simulink model "rendezvous_optimization_ALO"  (R2023a)
settings: Solver=VariableStepAuto  StartTime=0.0  StopTime=600  RelTol=1e-3
undefined symbols (not defined in the file): Ax, Ax_i, Ay, Ay_i, Az, Bx, Bx_i, By, By_i, Bz, Cx, Cx_i, Cy, Cy_i, Cz, IC_x_init, IC_y_init, juliandate, m0, mDot, OC_x_init, OC_y_init, OC_z_init, omega_T, Ve
(part 1 of 2)
settings Model: Creator=shubi  LastModifiedBy=shubi
settings SolverCC: ZeroCrossAlgorithm=Adaptive
settings DebuggingCC: AlgebraicLoopMsg=none  IgnoredZcDiagnostic=none

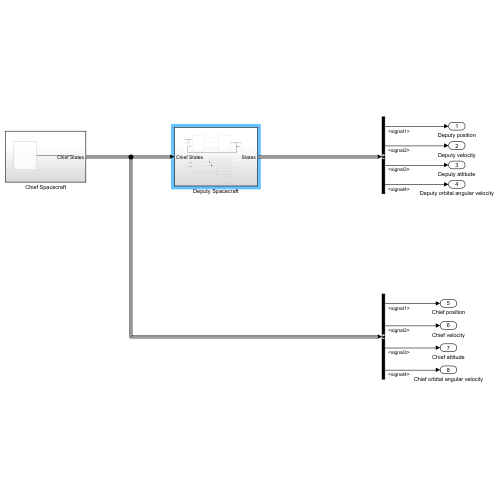
[thumbnail: Simulink's stored preview of the top-level diagram]
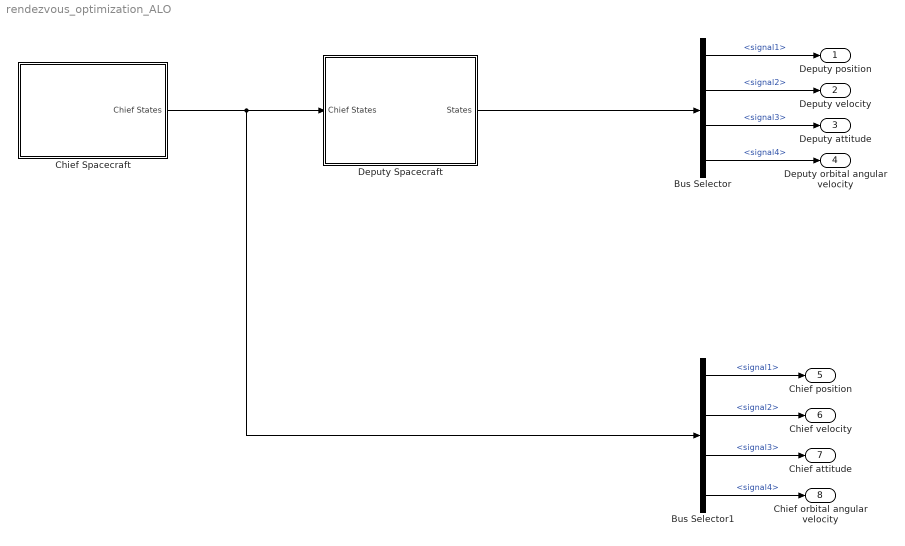
== system rendezvous_optimization_ALO ==
  Bus Selector : BusSelector  OutputSignals=signal1,signal2,signal3,signal4
  Bus Selector1 : BusSelector  OutputSignals=signal1,signal2,signal3,signal4
  Chief Spacecraft : Subsystem
  Deputy Spacecraft : Subsystem
  Deputy position : Outport
  Deputy velocity : Outport  Port=2
  Deputy attitude : Outport  Port=3
  Deputy orbital angular velocity : Outport  Port=4
  Chief position : Outport  Port=5
  Chief velocity : Outport  Port=6
  Chief attitude : Outport  Port=7
  Chief orbital angular velocity : Outport  Port=8
  wires:
  Bus Selector/4 -> Deputy orbital angular velocity/1  "<signal4>"
  Bus Selector1/4 -> Chief orbital angular velocity/1  "<signal4>"
  Bus Selector1/3 -> Chief attitude/1  "<signal3>"
  Bus Selector/2 -> Deputy velocity/1  "<signal2>"
  Bus Selector1/2 -> Chief velocity/1  "<signal2>"
  Bus Selector1/1 -> Chief position/1  "<signal1>"
  Chief Spacecraft/1(Chief States) -> Bus Selector1/1, Deputy Spacecraft/1(Chief States)
  Bus Selector/3 -> Deputy attitude/1  "<signal3>"
  Deputy Spacecraft/1(States) -> Bus Selector/1
  Bus Selector/1 -> Deputy position/1  "<signal1>"

== system rendezvous_optimization_ALO/Chief Spacecraft ==
  Spacecraft : Subsystem
  Chief States : Outport
  wires:
  Spacecraft/1(States) -> Chief States/1

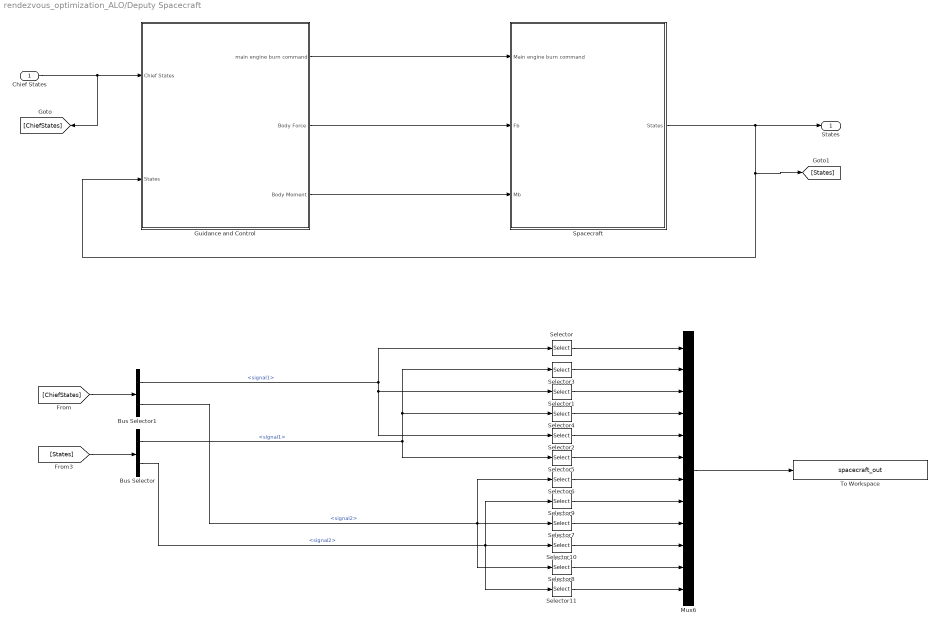
== system rendezvous_optimization_ALO/Deputy Spacecraft ==
  Chief States : Inport
  Bus Selector : BusSelector  OutputSignals=signal1,signal2
  Bus Selector1 : BusSelector  OutputSignals=signal1,signal2
  Guidance and Control : Subsystem
  Mux6 : Mux  Inputs=12
  Selector{,3,6,9} (4 alike) : Selector  InputPortWidth=3  IndexOptions=Index vector (dialog)  Indices=[1]  OutputSizes=1
  Selector{1,4,7,10} (4 alike) : Selector  InputPortWidth=3  IndexOptions=Index vector (dialog)  Indices=[2]  OutputSizes=1
  Selector{2,5,8,11} (4 alike) : Selector  InputPortWidth=3  IndexOptions=Index vector (dialog)  Indices=[3]  OutputSizes=1
  Spacecraft : Subsystem
  To Workspace : ToWorkspace  VariableName=spacecraft_out  SaveFormat=Timeseries  SampleTime=0.1
  States : Outport
  wires:
  Chief States/1 -> [ChiefStates], Guidance and Control/1(Chief States)
  Guidance and Control/3(Body Moment) -> Spacecraft/3(Mb)
  Guidance and Control/2(Body Force) -> Spacecraft/2(Fb)
  Guidance and Control/1(main engine burn command) -> Spacecraft/1(Main engine burn command)
  Spacecraft/1(States) -> [States], Guidance and Control/2(States), States/1
  Selector9/1 -> Mux6/8
  Selector2/1 -> Mux6/5
  Selector7/1 -> Mux6/9
  Selector11/1 -> Mux6/12
  Selector5/1 -> Mux6/6
  Mux6/1 -> To Workspace/1
  Selector4/1 -> Mux6/4
  Selector3/1 -> Mux6/2
  Selector8/1 -> Mux6/11
  [States] -> Bus Selector/1
  Selector1/1 -> Mux6/3
  Bus Selector/1 -> Selector5/1, Selector3/1, Selector4/1  "<signal1>"
  Selector10/1 -> Mux6/10
  Bus Selector/2 -> Selector9/1, Selector11/1, Selector10/1  "<signal2>"
  Bus Selector1/1 -> Selector/1, Selector2/1, Selector1/1  "<signal1>"
  Selector6/1 -> Mux6/7
  [ChiefStates] -> Bus Selector1/1
  Bus Selector1/2 -> Selector6/1, Selector8/1, Selector7/1  "<signal2>"
  Selector/1 -> Mux6/1

== system rendezvous_optimization_ALO/Chief Spacecraft/Spacecraft ==
  Bus Creator : BusCreator  Inputs=4
  Spacecraft Dynamics : SpacecraftDynamics  forcesIn=off  momentsIn=off  startDate=juliandate(2000, 1, 1, 12, 0, 0)  action=Error  mass=m0_C  emptyMass=m0-0.5  fullMass=m0  inertia=[600, 0, 0; 0, 500, 0; 0, 0, 550]  emptyInertia=[0.0058, 0, 0; 0, 0.0292, 0; 0, 0, 0.0292]  fullInertia=[0.0067, 0, 0; 0, 0.0333, 0; 0, 0, 0.0333]  useMassFlowRelativeVelocity=on  outputFuelStatus=off  semiMajorAxis=6878140  eccentricity=0  inclination=97.4065  raan=0  argPeriapsis=0  trueAnomaly=0  inertialPosition=[7229500.0, 4578700.0, -1432100.0]  attitude=[1, 0, 0,0]  attitudeRate=[-3, 2, 3]  useDrag=on  atmosSrc=Port  dragCoeffSrc=Port  dragAreaSrc=Port
  Terminator : Terminator
  atm. drag at 500km : Constant  Value=3e-12
  drag area : Constant
  drag coeff. : Constant  Value=2.2
  States : Outport
  wires:
  Spacecraft Dynamics/1 -> Bus Creator/1
  Spacecraft Dynamics/2 -> Bus Creator/2
  Spacecraft Dynamics/3 -> Bus Creator/3
  Spacecraft Dynamics/4 -> Bus Creator/4
  Bus Creator/1 -> States/1
  Spacecraft Dynamics/5 -> Terminator/1
  drag area/1 -> Spacecraft Dynamics/3
  drag coeff./1 -> Spacecraft Dynamics/2
  atm. drag at 500km/1 -> Spacecraft Dynamics/1

== system rendezvous_optimization_ALO/Deputy Spacecraft/Guidance and Control ==
  Chief States : Inport
  States : Inport  Port=2
  Control : Subsystem
  Guidance : Subsystem
  main engine burn command : Outport
  Body Force : Outport  Port=2
  Body Moment : Outport  Port=3
  wires:
  Chief States/1 -> Guidance/1(Chief States)
  Guidance/2(chief position) -> Control/1(chief position)
  Guidance/1(Main engine burn command) -> main engine burn command/1
  Control/1(Body Force) -> Body Force/1
  Control/2(Body Moment) -> Body Moment/1
  Guidance/3(chief velocity) -> Control/2(chief velocity)
  States/1 -> Control/3(States)

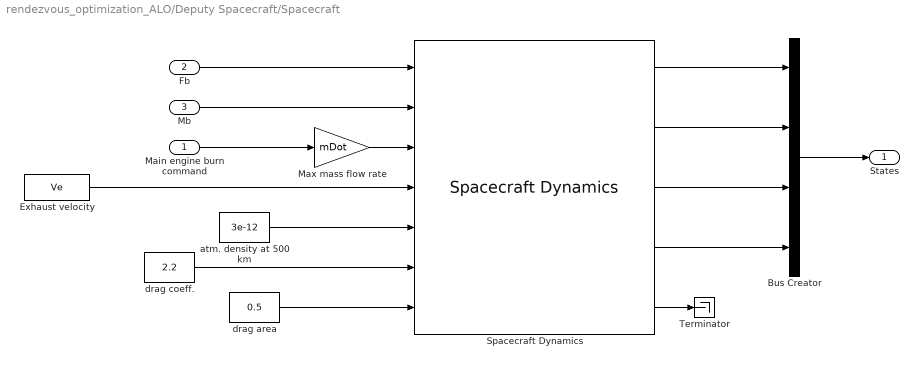
== system rendezvous_optimization_ALO/Deputy Spacecraft/Spacecraft ==
  Main engine burn command : Inport
  Fb : Inport  Port=2
  Mb : Inport  Port=3
  Bus Creator : BusCreator  Inputs=4
  Exhaust velocity : Constant  Value=Ve
  Max mass flow rate : Gain  Gain=mDot
  Spacecraft Dynamics : SpacecraftDynamics  startDate=juliandate(2000, 1, 1, 12, 0, 0)  massType=Simple variable  mass=m0  emptyMass=m0-0.5  fullMass=m0  emptyInertia=[0.0058, 0, 0; 0, 0.0292, 0; 0, 0, 0.0292]  fullInertia=[0.0067, 0, 0; 0, 0.0333, 0; 0, 0, 0.0333]  useMassFlowRelativeVelocity=on  outputFuelStatus=off  semiMajorAxis=a  eccentricity=e  inclination=inc  raan=Omega  argPeriapsis=omega  trueAnomaly=f  inertialPosition=[7229600.0,4578800.0,-1432100.0]  inertialVelocity=[-3823.0, 6844.2, 2978.8]  attitude=[1, 0, 0,0]  attitudeRate=[-0.8, 0.4, 0.8]  useDrag=on  atmosSrc=Port  dragCoeffSrc=Port  dragAreaSrc=Port
  Terminator : Terminator
  atm. density at 500 km : Constant  Value=3e-12
  drag area : Constant  Value=0.5
  drag coeff. : Constant  Value=2.2
  States : Outport
  wires:
  Mb/1 -> Spacecraft Dynamics/2
  Main engine burn command/1 -> Max mass flow rate/1
  Max mass flow rate/1 -> Spacecraft Dynamics/3
  Exhaust velocity/1 -> Spacecraft Dynamics/4
  Spacecraft Dynamics/1 -> Bus Creator/1
  Spacecraft Dynamics/3 -> Bus Creator/3
  Spacecraft Dynamics/4 -> Bus Creator/4
  Bus Creator/1 -> States/1
  Spacecraft Dynamics/5 -> Terminator/1
  Spacecraft Dynamics/2 -> Bus Creator/2
  Fb/1 -> Spacecraft Dynamics/1
  atm. density at 500 km/1 -> Spacecraft Dynamics/5
  drag area/1 -> Spacecraft Dynamics/7
  drag coeff./1 -> Spacecraft Dynamics/6

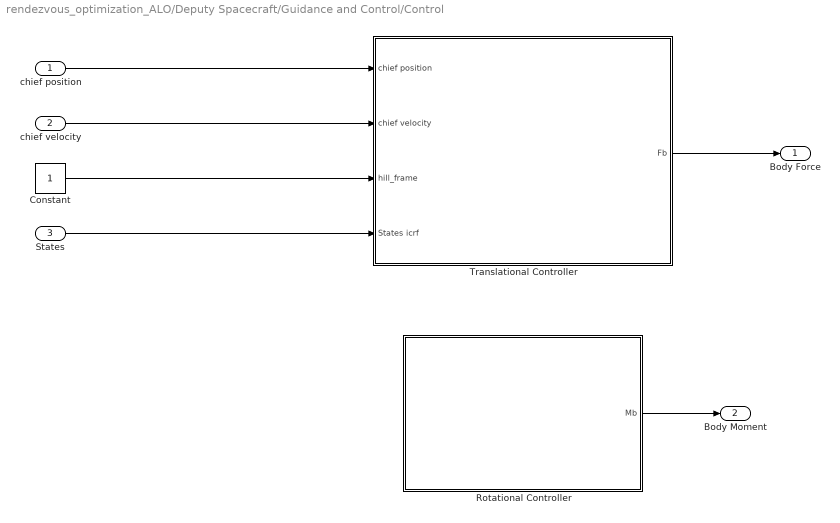
== system rendezvous_optimization_ALO/Deputy Spacecraft/Guidance and Control/Control ==
  chief position : Inport
  chief velocity : Inport  Port=2
  States : Inport  Port=3
  Constant : Constant
  Rotational Controller : Subsystem
  Translational Controller : Subsystem
  Body Force : Outport
  Body Moment : Outport  Port=2
  wires:
  Constant/1 -> Translational Controller/3(hill_frame)
  Rotational Controller/1(Mb) -> Body Moment/1
  chief position/1 -> Translational Controller/1(chief position)
  chief velocity/1 -> Translational Controller/2(chief velocity)
  States/1 -> Translational Controller/4(States icrf)
  Translational Controller/1(Fb) -> Body Force/1

== system rendezvous_optimization_ALO/Deputy Spacecraft/Guidance and Control/Guidance ==
  Chief States : Inport
  Enable Rendezvous : Constant
  Maneuver : Subsystem
  Terminator : Terminator
  Main engine burn command : Outport
  chief position : Outport  Port=2
  chief velocity : Outport  Port=3
  wires:
  Maneuver/1(Main engine burn command) -> Main engine burn command/1
  Chief States/1 -> Maneuver/1(Chief States)
  Enable Rendezvous/1 -> Maneuver/Enable
  Maneuver/2(chief position) -> chief position/1
  Maneuver/3(chief velocity) -> chief velocity/1
  Maneuver/4(Rotational Guidance) -> Terminator/1

== system rendezvous_optimization_ALO/Deputy Spacecraft/Guidance and Control/Control/Rotational Controller ==
  Moment : Constant  Value=[0,0,0]
  Mb : Outport
  wires:
  Moment/1 -> Mb/1

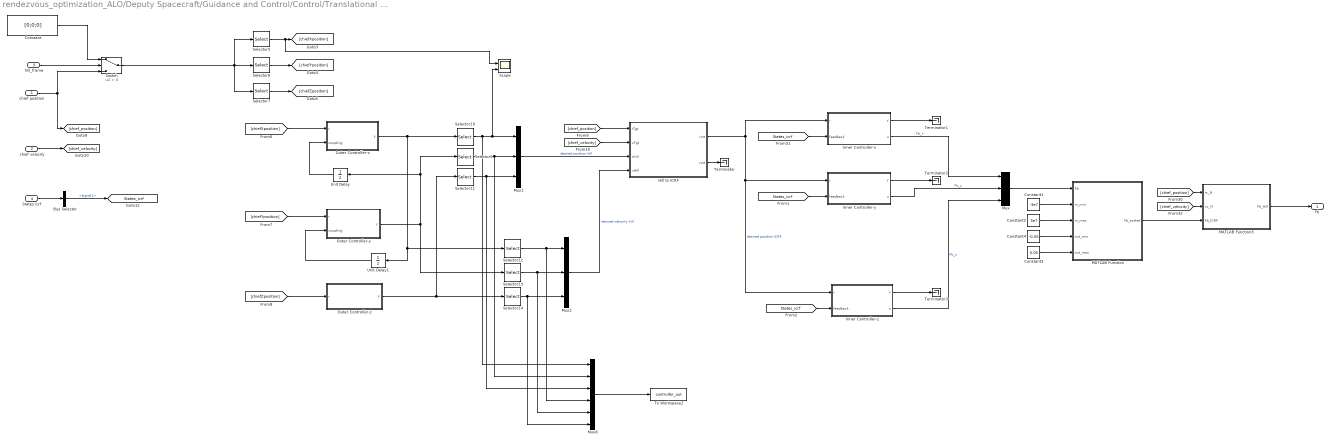
== system rendezvous_optimization_ALO/Deputy Spacecraft/Guidance and Control/Control/Translational Controller ==
  chief position : Inport
  chief velocity : Inport  Port=2
  hill_frame : Inport  Port=3
  States icrf : Inport  Port=4
  Bus Selector : BusSelector  OutputSignals=signal1
  Constant : Constant  Value=[0;0;0]
  Constant1 : Constant  Value=-3e7
  Constant2 : Constant  Value=3e7
  Constant3 : Constant  Value=0.05
  Constant4 : Constant  Value=-0.05
  Hill to ICRF : MATLAB Function  TreatAsAtomicUnit=on
  Inner Controller-x : Subsystem
  Inner Controller-y : Subsystem
  Inner Controller-z : Subsystem
  MATLAB Function : MATLAB Function  TreatAsAtomicUnit=on
  MATLAB Function3 : MATLAB Function  TreatAsAtomicUnit=on
  Mux : Mux  Inputs=3
  Mux1 : Mux  Inputs=3
  Mux2 : Mux  Inputs=3
  Mux8 : Mux  Inputs=6
  Outer Controller-x : Subsystem
  Outer Controller-y : Subsystem
  Outer Controller-z : Subsystem
  Scope : Scope  NumInputPorts=2
  Selector10 : Selector  InputPortWidth=2  IndexOptions=Index vector (dialog)  Indices=[1]  OutputSizes=1
  Selector11 : Selector  InputPortWidth=2  IndexOptions=Index vector (dialog)  Indices=[1]  OutputSizes=1
  Selector12 : Selector  InputPortWidth=2  IndexOptions=Index vector (dialog)  Indices=[2]  OutputSizes=1
  Selector13 : Selector  InputPortWidth=2  IndexOptions=Index vector (dialog)  Indices=[2]  OutputSizes=1
  Selector14 : Selector  InputPortWidth=2  IndexOptions=Index vector (dialog)  Indices=[2]  OutputSizes=1
  Selector5 : Selector  InputPortWidth=3  IndexOptions=Index vector (dialog)  Indices=[1]  OutputSizes=1
  Selector6 : Selector  InputPortWidth=3  IndexOptions=Index vector (dialog)  Indices=[2]  OutputSizes=1
  Selector7 : Selector  InputPortWidth=3  IndexOptions=Index vector (dialog)  Indices=[3]  OutputSizes=1
  Selector9 : Selector  InputPortWidth=2  IndexOptions=Index vector (dialog)  Indices=[1]  OutputSizes=1
  Switch : Switch  Criteria=u2 > Threshold  SaturateOnIntegerOverflow=off  InputSameDT=off
  Terminator{,1..3} (4 alike) : Terminator
  To Workspace2 : ToWorkspace  VariableName=controller_out  SaveFormat=Timeseries  SampleTime=0.1
  Unit Delay : UnitDelay  SampleTime=-1  HasFrameUpgradeWarning=on
  Unit Delay1 : UnitDelay  SampleTime=-1  HasFrameUpgradeWarning=on
  Fb : Outport
  tag scope: States_icrf=global
  wires:
  hill_frame/1 -> Switch/2
  Outer Controller-x/1(Y) -> Selector10/1, Unit Delay1/1, Selector12/1
  Unit Delay/1 -> Outer Controller-x/2(coupling)
  chief position/1 -> Switch/3, [chief_position]
  Outer Controller-y/1(Y) -> Selector9/1, Unit Delay/1, Selector13/1
  Unit Delay1/1 -> Outer Controller-y/2(coupling)
  Outer Controller-z/1(Y) -> Selector14/1, Selector11/1
  Constant/1 -> Switch/1
  Switch/1 -> Selector5/1, Selector7/1, Selector6/1
  Selector5/1 -> Scope/1, [chiefXposition]
  Selector6/1 -> [chiefYposition]
  Selector7/1 -> [chiefZposition]
  [chiefXposition] -> Outer Controller-x/1(r)
  [chiefYposition] -> Outer Controller-y/1(r)
  [chiefZposition] -> Outer Controller-z/1(r)
  chief velocity/1 -> [chief_velocity]
  [chief_position] -> Hill to ICRF/1(rTgt)
  [chief_velocity] -> Hill to ICRF/2(vTgt)
  Hill to ICRF/1(rInt) -> Inner Controller-z/1(r), Inner Controller-y/1(r), Inner Controller-x/1(r)  "desired position ICRF"
  Hill to ICRF/2(vInt) -> Terminator/1
  Selector10/1 -> Scope/2, Mux1/1, Mux8/1
  Selector11/1 -> Mux1/3, Mux8/3
  Mux1/1 -> Hill to ICRF/3(rHill)  "desired position hill"
  Selector13/1 -> Mux8/5, Mux2/2
  Selector14/1 -> Mux8/6, Mux2/3
  Mux2/1 -> Hill to ICRF/4(vHill)  "desired velocity hill"
  Selector9/1 -> Mux1/2, Mux8/2
  Mux8/1 -> To Workspace2/1
  Selector12/1 -> Mux2/1, Mux8/4
  Constant2/1 -> MATLAB Function/3(in_max)
  Constant4/1 -> MATLAB Function/4(out_min)
  MATLAB Function/1(Fb_scaled) -> MATLAB Function3/3(Fb_ICRF)
  [chief_velocity] -> MATLAB Function3/2(vc_N)
  Constant1/1 -> MATLAB Function/2(in_min)
  [chief_position] -> MATLAB Function3/1(rc_N)
  MATLAB Function3/1(Fb_Hill) -> Fb/1
  Mux/1 -> MATLAB Function/1(Fb)
  Constant3/1 -> MATLAB Function/5(out_max)
  Inner Controller-y/2(u) -> Mux/2  "Fb_y"
  States icrf/1 -> Bus Selector/1
  Bus Selector/1 -> [States_icrf]  "<signal1>"
  Inner Controller-z/2(u) -> Mux/3  "Fb_z"
  [States_icrf] -> Inner Controller-x/2(feedback)
  [States_icrf] -> Inner Controller-y/2(feedback)
  [States_icrf] -> Inner Controller-z/2(feedback)
  Inner Controller-x/2(u) -> Mux/1  "Fb_x"
  Inner Controller-x/1(Y) -> Terminator1/1
  Inner Controller-y/1(Y) -> Terminator2/1
  Inner Controller-z/1(Y) -> Terminator3/1

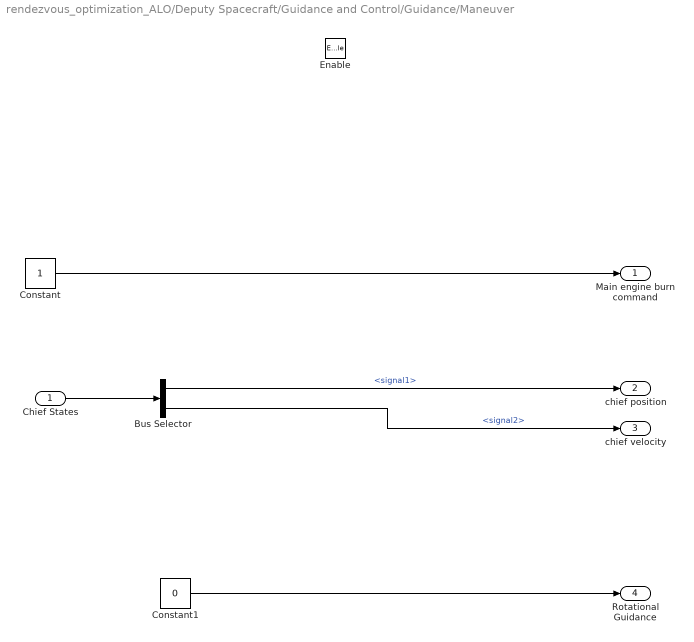
== system rendezvous_optimization_ALO/Deputy Spacecraft/Guidance and Control/Guidance/Maneuver ==
  Chief States : Inport
  Enable : EnablePort
  Bus Selector : BusSelector  OutputSignals=signal1,signal2
  Constant : Constant
  Constant1 : Constant  Value=0
  Main engine burn command : Outport
  chief position : Outport  Port=2
  chief velocity : Outport  Port=3
  Rotational Guidance : Outport  Port=4
  wires:
  Bus Selector/1 -> chief position/1  "<signal1>"
  Chief States/1 -> Bus Selector/1
  Constant/1 -> Main engine burn command/1
  Constant1/1 -> Rotational Guidance/1
  Bus Selector/2 -> chief velocity/1  "<signal2>"

== system rendezvous_optimization_ALO/Deputy Spacecraft/Guidance and Control/Control/Translational Controller/Inner Controller-x ==
  r : Inport
  feedback : Inport  Port=2
  Subsystem : Subsystem
  X-Axis : Subsystem
  Y : Outport
  u : Outport  Port=2
  wires:
  r/1 -> Subsystem/1(r)
  feedback/1 -> Subsystem/2(feedback)
  Subsystem/1(u) -> u/1, X-Axis/1(u)
  X-Axis/1(Y) -> Y/1

== system rendezvous_optimization_ALO/Deputy Spacecraft/Guidance and Control/Control/Translational Controller/Inner Controller-y ==
  r : Inport
  feedback : Inport  Port=2
  Subsystem : Subsystem
  Y-Axis : Subsystem
  Y : Outport
  u : Outport  Port=2
  wires:
  r/1 -> Subsystem/1(r)
  feedback/1 -> Subsystem/2(feedback)
  Subsystem/1(u) -> u/1, Y-Axis/1(u)
  Y-Axis/1(Y) -> Y/1

== system rendezvous_optimization_ALO/Deputy Spacecraft/Guidance and Control/Control/Translational Controller/Inner Controller-z ==
  r : Inport
  feedback : Inport  Port=2
  Subsystem : Subsystem
  Y-Axis : Subsystem
  Y : Outport
  u : Outport  Port=2
  wires:
  r/1 -> Subsystem/1(r)
  feedback/1 -> Subsystem/2(feedback)
  Subsystem/1(u) -> u/1, Y-Axis/1(u)
  Y-Axis/1(Y) -> Y/1

== system rendezvous_optimization_ALO/Deputy Spacecraft/Guidance and Control/Control/Translational Controller/Outer Controller-x ==
  r : Inport
  coupling : Inport  Port=2
  Controller-1 : Subsystem
  X-Axis : Subsystem
  Y : Outport
  wires:
  Controller-1/1(u) -> X-Axis/1(u)
  r/1 -> Controller-1/1(r)
  coupling/1 -> Controller-1/2(coupling)
  X-Axis/1(Y) -> Controller-1/3(x), Y/1  "feedback"

== system rendezvous_optimization_ALO/Deputy Spacecraft/Guidance and Control/Control/Translational Controller/Outer Controller-y ==
  r : Inport
  coupling : Inport  Port=2
  Controller-2 : Subsystem
  Y-Axis : Subsystem
  Y : Outport
  wires:
  r/1 -> Controller-2/1(r)
  coupling/1 -> Controller-2/2(coupling)
  Controller-2/1(u) -> Y-Axis/1(u)
  Y-Axis/1(Y1) -> Controller-2/3(x), Y/1  "feedback"

== system rendezvous_optimization_ALO/Deputy Spacecraft/Guidance and Control/Control/Translational Controller/Outer Controller-z ==
  r : Inport
  Controller-3 : Subsystem
  Z-Axis : Subsystem
  Y : Outport
  wires:
  r/1 -> Controller-3/1(r)
  Controller-3/1(u) -> Z-Axis/1(u)
  Z-Axis/1(Y) -> Controller-3/2(x), Y/1  "feedback"

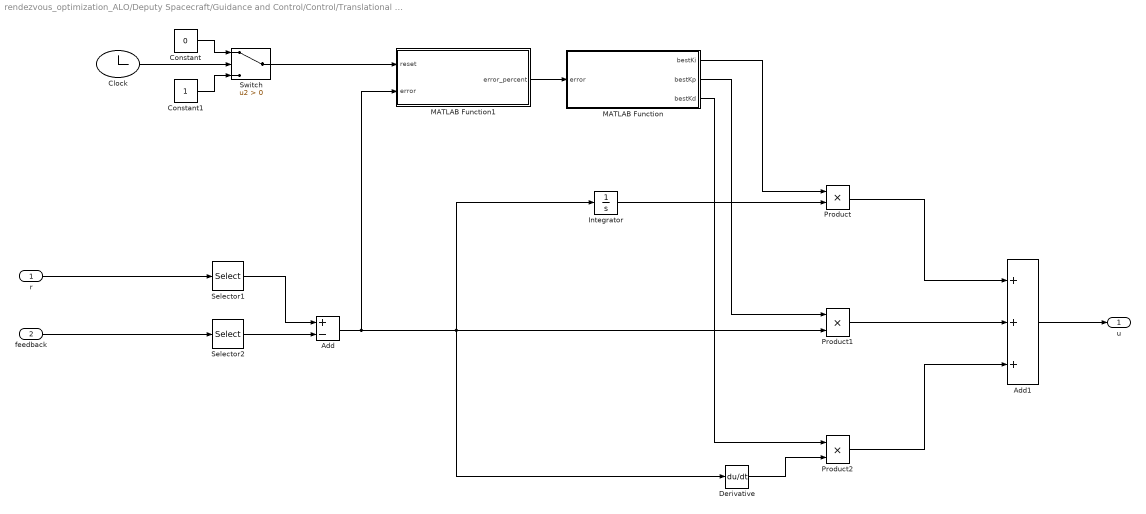
== system rendezvous_optimization_ALO/Deputy Spacecraft/Guidance and Control/Control/Translational Controller/Inner Controller-x/Subsystem ==
  r : Inport
  feedback : Inport  Port=2
  Add : Sum  Inputs=+-
  Add1 : Sum  Inputs=+++
  Clock : Clock
  Constant : Constant  Value=0
  Constant1 : Constant
  Derivative : Derivative
  Integrator : Integrator
  MATLAB Function : MATLAB Function  TreatAsAtomicUnit=on
  MATLAB Function1 : MATLAB Function  TreatAsAtomicUnit=on
  Product : Product
  Product1 : Product
  Product2 : Product
  Selector1 : Selector  InputPortWidth=3  IndexOptions=Index vector (dialog)  Indices=[1]  OutputSizes=1
  Selector2 : Selector  InputPortWidth=3  IndexOptions=Index vector (dialog)  Indices=[1]  OutputSizes=1
  Switch : Switch  Criteria=u2 > Threshold  SaturateOnIntegerOverflow=off  InputSameDT=off
  u : Outport
  wires:
  Integrator/1 -> Product/2
  Constant1/1 -> Switch/3
  Add1/1 -> u/1
  Add/1 -> MATLAB Function1/2(error), Product1/2, Integrator/1, Derivative/1
  Selector2/1 -> Add/2
  Product2/1 -> Add1/3
  Selector1/1 -> Add/1
  r/1 -> Selector1/1
  MATLAB Function1/1(error_percent) -> MATLAB Function/1(error)
  Clock/1 -> Switch/2
  Product1/1 -> Add1/2
  Product/1 -> Add1/1
  Constant/1 -> Switch/1
  feedback/1 -> Selector2/1
  Switch/1 -> MATLAB Function1/1(reset)
  Derivative/1 -> Product2/2
  MATLAB Function/1(bestKi) -> Product/1
  MATLAB Function/2(bestKp) -> Product1/1
  MATLAB Function/3(bestKd) -> Product2/1

== system rendezvous_optimization_ALO/Deputy Spacecraft/Guidance and Control/Control/Translational Controller/Inner Controller-x/X-Axis ==
  u : Inport
  state space : StateSpace  A=Ax_i  B=Bx_i  C=Cx_i  D=[0;0]  InitialCondition=IC_x_init  ParameterTunability=Unconstrained
  Y : Outport
  wires:
  u/1 -> state space/1
  state space/1 -> Y/1

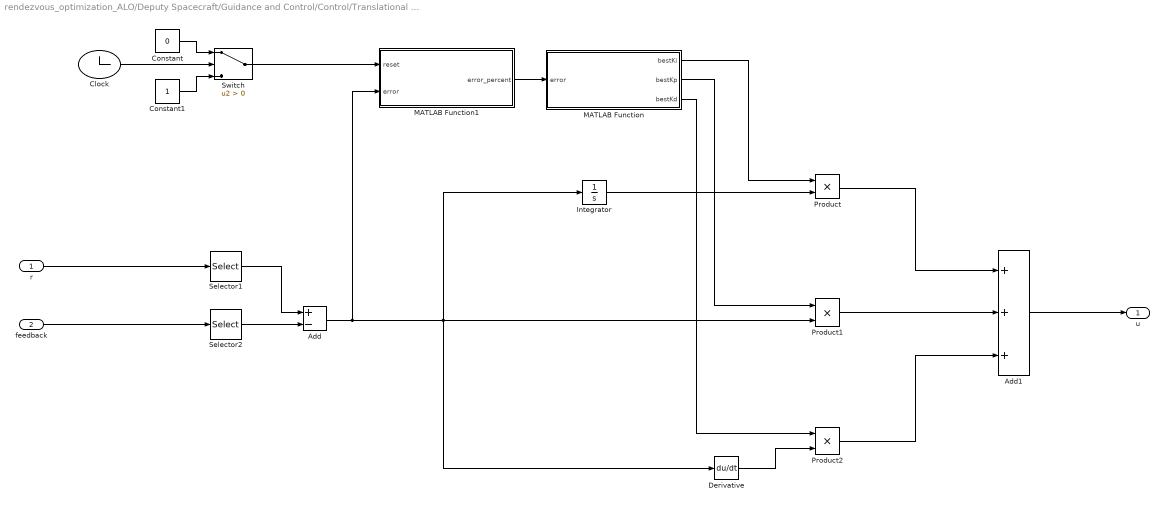
== system rendezvous_optimization_ALO/Deputy Spacecraft/Guidance and Control/Control/Translational Controller/Inner Controller-y/Subsystem ==
  r : Inport
  feedback : Inport  Port=2
  Add : Sum  Inputs=+-
  Add1 : Sum  Inputs=+++
  Clock : Clock
  Constant : Constant  Value=0
  Constant1 : Constant
  Derivative : Derivative
  Integrator : Integrator
  MATLAB Function : MATLAB Function  TreatAsAtomicUnit=on
  MATLAB Function1 : MATLAB Function  TreatAsAtomicUnit=on
  Product : Product
  Product1 : Product
  Product2 : Product
  Selector1 : Selector  InputPortWidth=3  IndexOptions=Index vector (dialog)  Indices=[2]  OutputSizes=1
  Selector2 : Selector  InputPortWidth=3  IndexOptions=Index vector (dialog)  Indices=[2]  OutputSizes=1
  Switch : Switch  Criteria=u2 > Threshold  SaturateOnIntegerOverflow=off  InputSameDT=off
  u : Outport
  wires:
  Add/1 -> MATLAB Function1/2(error), Product1/2, Integrator/1, Derivative/1
  Selector1/1 -> Add/1
  Integrator/1 -> Product/2
  feedback/1 -> Selector2/1
  Product2/1 -> Add1/3
  Clock/1 -> Switch/2
  r/1 -> Selector1/1
  Product1/1 -> Add1/2
  MATLAB Function1/1(error_percent) -> MATLAB Function/1(error)
  Constant/1 -> Switch/1
  Switch/1 -> MATLAB Function1/1(reset)
  Selector2/1 -> Add/2
  Product/1 -> Add1/1
  Add1/1 -> u/1
  Constant1/1 -> Switch/3
  Derivative/1 -> Product2/2
  MATLAB Function/1(bestKi) -> Product/1
  MATLAB Function/2(bestKp) -> Product1/1
  MATLAB Function/3(bestKd) -> Product2/1

== system rendezvous_optimization_ALO/Deputy Spacecraft/Guidance and Control/Control/Translational Controller/Inner Controller-y/Y-Axis ==
  u : Inport
  state space : StateSpace  A=Ay_i  B=By_i  C=Cy_i  D=[0;0]  InitialCondition=IC_y_init  ParameterTunability=Unconstrained
  Y : Outport
  wires:
  u/1 -> state space/1
  state space/1 -> Y/1

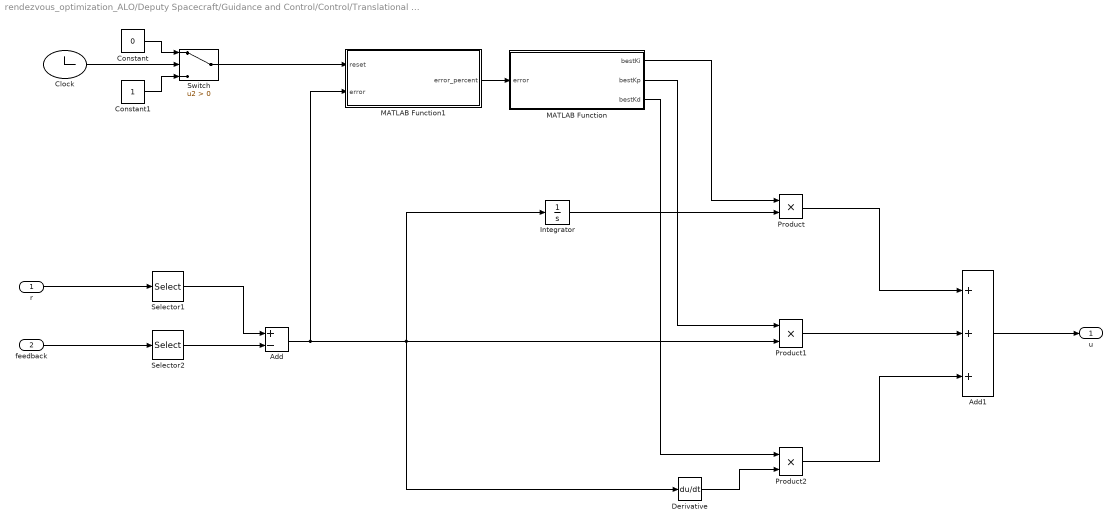
== system rendezvous_optimization_ALO/Deputy Spacecraft/Guidance and Control/Control/Translational Controller/Inner Controller-z/Subsystem ==
  r : Inport
  feedback : Inport  Port=2
  Add : Sum  Inputs=+-
  Add1 : Sum  Inputs=+++
  Clock : Clock
  Constant : Constant  Value=0
  Constant1 : Constant
  Derivative : Derivative
  Integrator : Integrator
  MATLAB Function : MATLAB Function  TreatAsAtomicUnit=on
  MATLAB Function1 : MATLAB Function  TreatAsAtomicUnit=on
  Product : Product
  Product1 : Product
  Product2 : Product
  Selector1 : Selector  InputPortWidth=3  IndexOptions=Index vector (dialog)  Indices=[3]  OutputSizes=1
  Selector2 : Selector  InputPortWidth=3  IndexOptions=Index vector (dialog)  Indices=[3]  OutputSizes=1
  Switch : Switch  Criteria=u2 > Threshold  SaturateOnIntegerOverflow=off  InputSameDT=off
  u : Outport
  wires:
  feedback/1 -> Selector2/1
  Add/1 -> MATLAB Function1/2(error), Product1/2, Integrator/1, Derivative/1
  MATLAB Function1/1(error_percent) -> MATLAB Function/1(error)
  Selector1/1 -> Add/1
  Derivative/1 -> Product2/2
  Integrator/1 -> Product/2
  Product1/1 -> Add1/2
  Clock/1 -> Switch/2
  Selector2/1 -> Add/2
  Switch/1 -> MATLAB Function1/1(reset)
  Add1/1 -> u/1
  Product/1 -> Add1/1
  Constant/1 -> Switch/1
  Constant1/1 -> Switch/3
  Product2/1 -> Add1/3
  r/1 -> Selector1/1
  MATLAB Function/1(bestKi) -> Product/1
  MATLAB Function/2(bestKp) -> Product1/1
  MATLAB Function/3(bestKd) -> Product2/1

== system rendezvous_optimization_ALO/Deputy Spacecraft/Guidance and Control/Control/Translational Controller/Inner Controller-z/Y-Axis ==
  u : Inport
  state space : StateSpace  A=Ay_i  B=By_i  C=Cy_i  D=[0;0]  InitialCondition=IC_y_init  ParameterTunability=Unconstrained
  Y : Outport
  wires:
  u/1 -> state space/1
  state space/1 -> Y/1

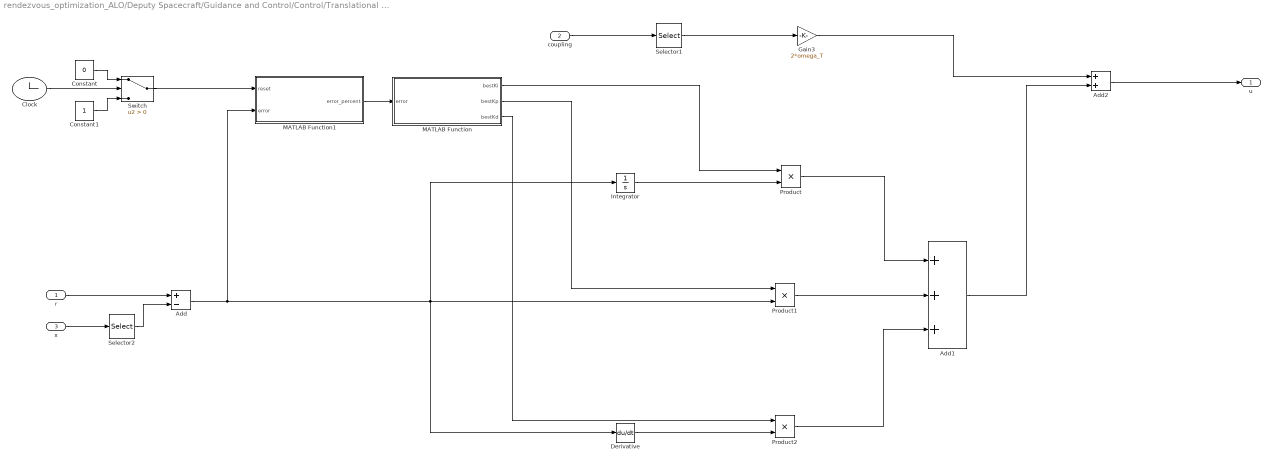
== system rendezvous_optimization_ALO/Deputy Spacecraft/Guidance and Control/Control/Translational Controller/Outer Controller-x/Controller-1 ==
  r : Inport
  coupling : Inport  Port=2
  x : Inport  Port=3
  Add : Sum  Inputs=+-
  Add1 : Sum  Inputs=+++
  Add2 : Sum
  Clock : Clock
  Constant : Constant  Value=0
  Constant1 : Constant
  Derivative : Derivative
  Gain3 : Gain  Gain=2*omega_T
  Integrator : Integrator
  MATLAB Function : MATLAB Function  TreatAsAtomicUnit=on
  MATLAB Function1 : MATLAB Function  TreatAsAtomicUnit=on
  Product : Product
  Product1 : Product
  Product2 : Product
  Selector1 : Selector  InputPortWidth=2  IndexOptions=Index vector (dialog)  Indices=[2]  OutputSizes=1
  Selector2 : Selector  InputPortWidth=2  IndexOptions=Index vector (dialog)  Indices=[1]  OutputSizes=1
  Switch : Switch  Criteria=u2 > Threshold  SaturateOnIntegerOverflow=off  InputSameDT=off
  u : Outport
  wires:
  r/1 -> Add/1
  coupling/1 -> Selector1/1
  Add2/1 -> u/1
  Product/1 -> Add1/1
  Selector2/1 -> Add/2
  Integrator/1 -> Product/2
  Product2/1 -> Add1/3
  Add1/1 -> Add2/2
  Product1/1 -> Add1/2
  x/1 -> Selector2/1
  Gain3/1 -> Add2/1
  Derivative/1 -> Product2/2
  Constant/1 -> Switch/1
  Clock/1 -> Switch/2
  Switch/1 -> MATLAB Function1/1(reset)
  Add/1 -> MATLAB Function1/2(error), Derivative/1, Integrator/1, Product1/2
  Constant1/1 -> Switch/3
  MATLAB Function1/1(error_percent) -> MATLAB Function/1(error)
  Selector1/1 -> Gain3/1
  MATLAB Function/1(bestKi) -> Product/1
  MATLAB Function/2(bestKp) -> Product1/1
  MATLAB Function/3(bestKd) -> Product2/1

== system rendezvous_optimization_ALO/Deputy Spacecraft/Guidance and Control/Control/Translational Controller/Outer Controller-x/X-Axis ==
  u : Inport
  state space : StateSpace  A=Ax  B=Bx  C=Cx  D=[0;0]  InitialCondition=OC_x_init  ParameterTunability=Unconstrained
  Y : Outport
  wires:
  u/1 -> state space/1
  state space/1 -> Y/1

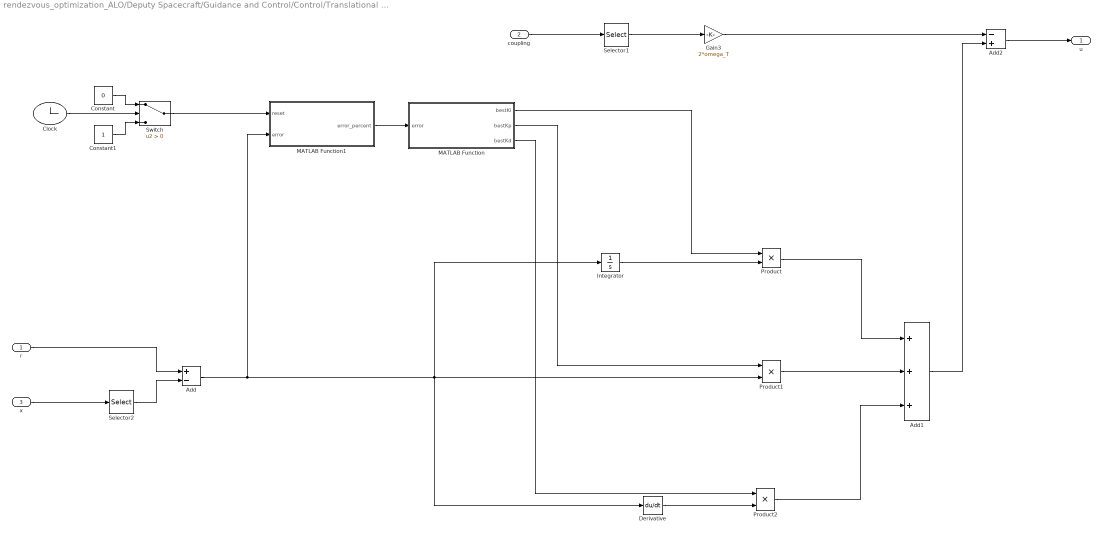
== system rendezvous_optimization_ALO/Deputy Spacecraft/Guidance and Control/Control/Translational Controller/Outer Controller-y/Controller-2 ==
  r : Inport
  coupling : Inport  Port=2
  x : Inport  Port=3
  Add : Sum  Inputs=+-
  Add1 : Sum  Inputs=+++
  Add2 : Sum  Inputs=-+
  Clock : Clock
  Constant : Constant  Value=0
  Constant1 : Constant
  Derivative : Derivative
  Gain3 : Gain  Gain=2*omega_T
  Integrator : Integrator
  MATLAB Function : MATLAB Function  TreatAsAtomicUnit=on
  MATLAB Function1 : MATLAB Function  TreatAsAtomicUnit=on
  Product : Product
  Product1 : Product
  Product2 : Product
  Selector1 : Selector  InputPortWidth=2  IndexOptions=Index vector (dialog)  Indices=[2]  OutputSizes=1
  Selector2 : Selector  InputPortWidth=2  IndexOptions=Index vector (dialog)  Indices=[1]  OutputSizes=1
  Switch : Switch  Criteria=u2 > Threshold  SaturateOnIntegerOverflow=off  InputSameDT=off
  u : Outport
  wires:
  Product/1 -> Add1/1
  x/1 -> Selector2/1
  Integrator/1 -> Product/2
  coupling/1 -> Selector1/1
  Gain3/1 -> Add2/1
  Product2/1 -> Add1/3
  Selector2/1 -> Add/2
  r/1 -> Add/1
  Derivative/1 -> Product2/2
  Add2/1 -> u/1
  Add1/1 -> Add2/2
  Product1/1 -> Add1/2
  Constant1/1 -> Switch/3
  Switch/1 -> MATLAB Function1/1(reset)
  Constant/1 -> Switch/1
  Add/1 -> MATLAB Function1/2(error), Derivative/1, Integrator/1, Product1/2
  Clock/1 -> Switch/2
  MATLAB Function1/1(error_percent) -> MATLAB Function/1(error)
  Selector1/1 -> Gain3/1
  MATLAB Function/1(bestKi) -> Product/1
  MATLAB Function/2(bestKp) -> Product1/1
  MATLAB Function/3(bestKd) -> Product2/1

== system rendezvous_optimization_ALO/Deputy Spacecraft/Guidance and Control/Control/Translational Controller/Outer Controller-y/Y-Axis ==
  u : Inport
  state space : StateSpace  A=Ay  B=By  C=Cy  D=[0;0]  InitialCondition=OC_y_init  ParameterTunability=Unconstrained
  Y1 : Outport
  wires:
  u/1 -> state space/1
  state space/1 -> Y1/1

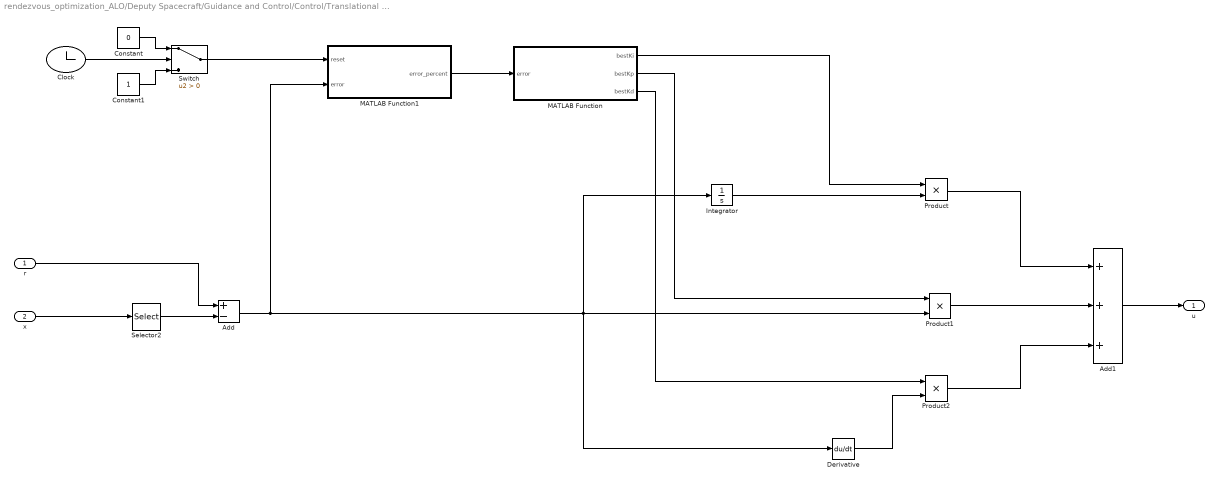
== system rendezvous_optimization_ALO/Deputy Spacecraft/Guidance and Control/Control/Translational Controller/Outer Controller-z/Controller-3 ==
  r : Inport
  x : Inport  Port=2
  Add : Sum  Inputs=+-
  Add1 : Sum  Inputs=+++
  Clock : Clock
  Constant : Constant  Value=0
  Constant1 : Constant
  Derivative : Derivative
  Integrator : Integrator
  MATLAB Function : MATLAB Function  TreatAsAtomicUnit=on
  MATLAB Function1 : MATLAB Function  TreatAsAtomicUnit=on
  Product : Product
  Product1 : Product
  Product2 : Product
  Selector2 : Selector  InputPortWidth=2  IndexOptions=Index vector (dialog)  Indices=[1]  OutputSizes=1
  Switch : Switch  Criteria=u2 > Threshold  SaturateOnIntegerOverflow=off  InputSameDT=off
  u : Outport
  wires:
  r/1 -> Add/1
  Selector2/1 -> Add/2
  x/1 -> Selector2/1
  Add1/1 -> u/1
  Integrator/1 -> Product/2
  Product/1 -> Add1/1
  Product1/1 -> Add1/2
  Derivative/1 -> Product2/2
  Product2/1 -> Add1/3
  Add/1 -> MATLAB Function1/2(error), Integrator/1, Product1/2, Derivative/1
  Constant1/1 -> Switch/3
  Switch/1 -> MATLAB Function1/1(reset)
  Constant/1 -> Switch/1
  Clock/1 -> Switch/2
  MATLAB Function1/1(error_percent) -> MATLAB Function/1(error)
  MATLAB Function/1(bestKi) -> Product/1
  MATLAB Function/2(bestKp) -> Product1/1
  MATLAB Function/3(bestKd) -> Product2/1

== system rendezvous_optimization_ALO/Deputy Spacecraft/Guidance and Control/Control/Translational Controller/Outer Controller-z/Z-Axis ==
  u : Inport
  state space : StateSpace  A=Az  B=Bz  C=Cz  D=[0;0]  InitialCondition=OC_z_init  ParameterTunability=Unconstrained
  Y : Outport
  wires:
  u/1 -> state space/1
  state space/1 -> Y/1

== matlab function rendezvous_optimization_ALO/Deputy Spacecraft/Guidance and Control/Control/Translational Controller/Outer Controller-y/Controller-2/MATLAB Function1 ==
  settings: updateMethod=DISCRETE
  data: reset input; error_percent output; error input
function error_percent = computeScheduledGain(reset,error)
% Compute gain based on percentage error using 1D look-up style logic
%
% Inputs:
%   r_des     : 3x1 desired position vector
%   r_current : 3x1 current position vector (from chaser)
%   r_init    : 3x1 initial position vector
%
% Output:
%   gain      : scalar scheduled gain

    persistent max_error;

    if reset || isempty(max_error)
        max_error = norm(error);  % store initial max error
    end
    
    e_now = norm(error);       % current error
    error_percent = (e_now / max_error)*100;       % normalized error: [0, 1]

   
end

== matlab function rendezvous_optimization_ALO/Deputy Spacecraft/Guidance and Control/Control/Translational Controller/Outer Controller-z/Controller-3/MATLAB Function1 ==
  settings: updateMethod=DISCRETE
  data: reset input; error_percent output; error input
function error_percent = computeScheduledGain(reset,error)
% Compute gain based on percentage error using 1D look-up style logic
%
% Inputs:
%   r_des     : 3x1 desired position vector
%   r_current : 3x1 current position vector (from chaser)
%   r_init    : 3x1 initial position vector
%
% Output:
%   gain      : scalar scheduled gain

    persistent max_error;

    if reset || isempty(max_error)
        max_error = norm(error);  % store initial max error
    end
    
    e_now = norm(error);       % current error
    error_percent = (e_now / max_error)*100;       % normalized error: [0, 1]

   
end

== matlab function rendezvous_optimization_ALO/Deputy Spacecraft/Guidance and Control/Control/Translational Controller/Hill to ICRF ==
  data: rTgt input; rInt output; vTgt input; rHill input; vHill input; vInt output
function [rInt,vInt] = Hill2ECI_Vectorized(rTgt,vTgt,rHill,vHill)
%% Purpose:
% Convert those position (rHill) and velocity (vHill) values back into an
% ECI coordinate frame of reference using the reference satellite
% (rTgt,vTgt) position and velocity data.
%
%% Inputs:
%rTgt                       [3 x N]                 ECI Position vector of
%                                                   reference frame (km)
%
%vTgt                       [3 x N]                 ECI Velocity vector of
%                                                   reference frame (km/s)
%
%rHill                      [3 x N]                 Hill's relative
%                                                   position vector (km)
%
%vHill                      [3 x N]                 Hill's relative
%                                                   velocity vector (km/s)
%
%
%
%% Outputs:
%rInt                       [3 x N]
%
%vInt                       [3 x N]
%
%
% References:
% Vallado 2007.
% Programed by Darin C Koblick 11/30/2012

rTgt = rTgt *0.001;
vTgt = vTgt*0.001;
rHill = rHill*0.001;
vHill  =vHill*0.001;
%% Begin Code Sequence
%Declare Local Functions
rTgtMag = sqrt(sum(rTgt.^2,1));
vTgtMag = sqrt(sum(vTgt.^2,1));
matrixMultiply = @(x,y)permute(cat(2,sum(permute(x(1,:,:),[3 2 1]).*permute(y,[2 1]),2), ...
                                     sum(permute(x(2,:,:),[3 2 1]).*permute(y,[2 1]),2), ...
                                     sum(permute(x(3,:,:),[3 2 1]).*permute(y,[2 1]),2)),[2 1]);
%Find the RSW matrix from the target ECI positions
RSW = ECI2RSW(rTgt,vTgt); rIntMag = rTgtMag + rHill(1,:);
%Compute rotation angles to go from tgt to interceptor
lambda_int = rHill(2,:)./rTgtMag; phi_int = sin(rHill(3,:)./rTgtMag);
CLI = cos(lambda_int); SLI = sin(lambda_int); CPI = cos(phi_int); SPI = sin(phi_int);
%find rotation matrix to go from rsw to SEZ of inerceptor
RSW_SEZ = zeros(3,3,size(rTgt,2));
RSW_SEZ(1,1,:) = SPI.*CLI;  RSW_SEZ(1,2,:) = SPI.*SLI; RSW_SEZ(1,3,:) = -CPI;
RSW_SEZ(2,1,:) = -SLI;      RSW_SEZ(2,2,:) = CLI;      RSW_SEZ(3,1,:) = CPI.*CLI;
                            RSW_SEZ(3,2,:) = CPI.*SLI; RSW_SEZ(3,3,:) = SPI;
%Find velocity component positions by using angular rates in SEZ frame
vIntSEZ = cat(1,-rIntMag.*vHill(3,:)./rTgtMag, ...
                 rIntMag.*(vHill(2,:)./rTgtMag + vTgtMag./rTgtMag).*CPI, ...
                 vHill(1,:));
vInt = matrixMultiply(permute(RSW,[2 1 3]), ...
       matrixMultiply(permute(RSW_SEZ,[2 1 3]), ...
       vIntSEZ));
%Find the position components
rIntRSW = bsxfun(@times,rIntMag,cat(1,CPI.*CLI, ...
                                      CPI.*SLI, ...
                                      SPI));
rInt = matrixMultiply(permute(RSW,[2 1 3]),rIntRSW); 

rInt = rInt *1000;
vInt = vInt*1000;
end

function [T,rRSW,vRSW] = ECI2RSW(rECI,vECI)
%% Purpose:
%Convert ECI Coordinates to RSW Coordinates, also, return the
%transformation matrix T in which to take a given set of coordinates in ECI
%and convert them using the same RSW reference frame.
%
%% Inputs:
% rECI              [3 x N]                     ECI position Coordinates in
%                                               km
%
% vECI              [3 x N]                     ECI velocity Coordinates in
%                                               km/s
%
%% Outputs:
% T                 [3 x 3 x N]                 Transformation matrix
%                                               necessary to go from
%                                               rECI -> rRSW
%
% rRSW              [3 x N]                     RSW Position Coordinates
%                                               km
%
% vRSW              [3 x N]                     RSW Velocity Coordinates
%                                               km/s
%
%% References:
% Vallado pg. 173
% Vallado rv2rsw.m code dated 06/09/2002
%
%Programmed by: Darin C Koblick                 11/29/2012
%% Begin Code Sequence
if nargin == 0
    rECI =  repmat([6968.1363,1,2]',[1 10]);
    vECI =  repmat([3,7.90536615282099,4]',[1 10]);
    [T,rRSW,vRSW] = ECI2RSW(rECI,vECI);
    return;
end
%Declared Internal function set:
unitv = @(x)bsxfun(@rdivide,x,sqrt(sum(x.^2,1)));
matrixMultiply = @(x,y)permute(cat(2,sum(permute(x(1,:,:),[3 2 1]).*permute(y,[2 1]),2), ...
                                     sum(permute(x(2,:,:),[3 2 1]).*permute(y,[2 1]),2), ...
                                     sum(permute(x(3,:,:),[3 2 1]).*permute(y,[2 1]),2)),[2 1]);
%Find the Radial component of the RIC position vector
rvec = unitv(rECI);
%Find the cross-track component of the RIC position vector
wvec = unitv(cross(rECI,vECI));
%Find the along-track component of the RIC position vector
svec = unitv(cross(wvec,rvec));
%Create the transformation matrix from ECI to RSW
T = NaN(3,3,size(rECI,2));
T(1,1,:) = rvec(1,:); T(1,2,:) = rvec(2,:); T(1,3,:) = rvec(3,:);
T(2,1,:) = svec(1,:); T(2,2,:) = svec(2,:); T(2,3,:) = svec(3,:);
T(3,1,:) = wvec(1,:); T(3,2,:) = wvec(2,:); T(3,3,:) = wvec(3,:);
%Find the position and velocity vectors in the RSW reference frame!
rRSW = matrixMultiply(T,rECI);
vRSW = matrixMultiply(T,vECI);
end

== matlab function rendezvous_optimization_ALO/Deputy Spacecraft/Guidance and Control/Control/Translational Controller/Inner Controller-x/Subsystem/MATLAB Function1 ==
  settings: updateMethod=DISCRETE
  data: reset input; error_percent output; error input
function error_percent = computeScheduledGain(reset,error)
% Compute gain based on percentage error using 1D look-up style logic
%
% Inputs:
%   r_des     : 3x1 desired position vector
%   r_current : 3x1 current position vector (from chaser)
%   r_init    : 3x1 initial position vector
%
% Output:
%   gain      : scalar scheduled gain

    persistent max_error;

    if reset || isempty(max_error)
        max_error = norm(error);  % store initial max error
    end
    
    e_now = norm(error);       % current error
    error_percent = (e_now / max_error)*100;       % normalized error: [0, 1]

   
end

== matlab function rendezvous_optimization_ALO/Deputy Spacecraft/Guidance and Control/Control/Translational Controller/Inner Controller-y/Subsystem/MATLAB Function1 ==
  settings: updateMethod=DISCRETE
  data: reset input; error_percent output; error input
function error_percent = computeScheduledGain(reset,error)
% Compute gain based on percentage error using 1D look-up style logic
%
% Inputs:
%   r_des     : 3x1 desired position vector
%   r_current : 3x1 current position vector (from chaser)
%   r_init    : 3x1 initial position vector
%
% Output:
%   gain      : scalar scheduled gain

    persistent max_error;

    if reset || isempty(max_error)
        max_error = norm(error);  % store initial max error
    end
    
    e_now = norm(error);       % current error
    error_percent = (e_now / max_error)*100;       % normalized error: [0, 1]

   
end

== matlab function rendezvous_optimization_ALO/Deputy Spacecraft/Guidance and Control/Control/Translational Controller/Inner Controller-z/Subsystem/MATLAB Function1 ==
  settings: updateMethod=DISCRETE
  data: reset input; error_percent output; error input
function error_percent = computeScheduledGain(reset,error)
% Compute gain based on percentage error using 1D look-up style logic
%
% Inputs:
%   r_des     : 3x1 desired position vector
%   r_current : 3x1 current position vector (from chaser)
%   r_init    : 3x1 initial position vector
%
% Output:
%   gain      : scalar scheduled gain

    persistent max_error;

    if reset || isempty(max_error)
        max_error = norm(error);  % store initial max error
    end
    
    e_now = norm(error);       % current error
    error_percent = (e_now / max_error)*100;       % normalized error: [0, 1]

   
end

== matlab function rendezvous_optimization_ALO/Deputy Spacecraft/Guidance and Control/Control/Translational Controller/Inner Controller-y/Subsystem/MATLAB Function ==
  settings: updateMethod=DISCRETE
  data: bestKi output; bestKp output; bestKd output; error input
function [bestKi,bestKp,bestKd] = antlion(error)
% antlion  Tune PID gains [Kp,Ki,Kd] via Ant Lion Optimizer
%
%   sys  = your state‐space or transfer‐function plant
%   [bestKp,bestKi,bestKd] = antlion(sys)

  %% ALO parameters
  nAnt     = 20;          
  Max_iter = 100;
  dim = 3;
  lb       = [0   0   0];  
  ub       = [10 5 10];  

  %% Run Ant Lion Optimizer
  %bestGains = runALO(error, nAnt, Max_iter, lb, ub);
  %bestKp = bestGains(1);
  %bestKi = bestGains(2);
  %bestKd = bestGains(3);
  %fprintf('Optimized gains: Kp=%.4f, Ki=%.4f, Kd=%.4f\n', ...
  %        bestKp, bestKi, bestKd);

   % Initialization
  antlions = rand(nAnt,dim) .* (ub - lb) + lb;
  ants     = zeros(nAnt, dim);
  fitAL    = inf(nAnt,1);
  
  % Evaluate initial fitness
  for i = 1:nAnt
      fitAL(i) = error;
  end
  elite = antlions(1,:);  % Initial elite antlion
  bestScore = fitAL(1);
  % Main loop
  for iter = 1:Max_iter
      % Update elite antlion
      [currBest, idx] = min(fitAL);
      if currBest < bestScore
          elite = antlions(idx,:);
          bestScore = currBest;
      end
      % Adaptive narrowing boundaries
      I = 10^iter/Max_iter;
      for i = 1:nAnt
          % Roulette wheel selection
          selectedAL = antlions(RouletteWheelSelection(1./(fitAL + eps)), :);
          % Random walk around selectedAL and elite
          RW1 = createRandomWalk(iter, Max_iter, lb, ub);
          RW2 = createRandomWalk(iter, Max_iter, lb, ub);
          ants(i,:) = (RW1 + RW2) / 2;
          % Bounds check
          ants(i,:) = max(min(ants(i,:), ub), lb);
      end
      % Evaluate ants
      fitAnts = inf(nAnt,1);
      for i = 1:nAnt
          fitAnts(i) = error;
      end
      % Merge and select next gen
      allPop = [antlions; ants];
      allFit = [fitAL; fitAnts];
      [allFit, idx] = sort(allFit);
      antlions = allPop(idx(1:nAnt), :);
      fitAL    = allFit(1:nAnt);
  end
  bestKp = elite(1); bestKi = elite(2); bestKd = elite(3);
end

%% Helper: Random walk (normalized)
function RW = createRandomWalk(iter, Max_iter, lb, ub)
    steps = 2*(rand(1,Max_iter)>0.5) - 1;
    walk = cumsum(steps);
    walk = (walk - min(walk)) / max(1e-6, max(walk) - min(walk)); % normalized
    RW = lb + walk(iter) .* (ub - lb);
end

%% Helper: Roulette Wheel
function idx = RouletteWheelSelection(probabilities)
    C = cumsum(probabilities / sum(probabilities));
    r = rand;
    idx = find(C >= r, 1, 'first');
end



%function bestGains = runALO(error, nAnt, Max_iter, lb, ub)
%  dim      = numel(lb);
%  antlions = rand(nAnt,dim).*(ub-lb)+lb;
%  ants      = zeros(nAnt,dim);
%  fitAL     = zeros(nAnt,1);
%
%  % Evaluate initial fitness
%  for i=1:nAnt
%    fitAL(i) = error;
%  end
%
%  for iter=1:Max_iter
%    % Roulette wheel selection
%    invFit = 1./(fitAL+eps);
%    P      = invFit/sum(invFit);
%    C      = cumsum(P);
%
%    % Move ants
%    for i=1:nAnt
%      r   = rand;
%      sel = find(C>=r,1);
%      AL  = antlions(sel,:);    % 1×3
%
%      RW = zeros(1,dim);
%      for d=1:dim
%        RW(d) = randomWalk(iter,Max_iter, lb(d), ub(d));
%      end
%
%      ants(i,:) = max(min(AL+RW, ub), lb);
%    end
%
%    % Evaluate ants
%    fitAnts = zeros(nAnt,1);
%    for i=1:nAnt
%      fitAnts(i) = error;
%    end
%
%    % Combine and select next generation antlions
%    allPop   = [antlions; ants];
%    allFit   = [fitAL; fitAnts];
%    [allFit, idx] = sort(allFit);
%    antlions = allPop(idx(1:nAnt), :);
%    fitAL    = allFit(1:nAnt);
%  end
%
%  bestGains = antlions(1,:);
%end
%
%
%function val = randomWalk(iter, Max_iter, lb, ub)
%  steps = 2*(rand(1,Max_iter)>0.5)-1;
%  walk  = cumsum(steps);
%  mn    = min(walk); mx = max(walk);
%  if mx>mn
%    normWalk = (walk-mn)/(mx-mn);
%  else
%    normWalk = zeros(size(walk));
%  end
%  val = lb + normWalk(iter)*(ub-lb);
%end

== matlab function rendezvous_optimization_ALO/Deputy Spacecraft/Guidance and Control/Control/Translational Controller/Inner Controller-z/Subsystem/MATLAB Function ==
  settings: updateMethod=DISCRETE
  data: bestKi output; bestKp output; bestKd output; error input
function [bestKi,bestKp,bestKd] = antlion(error)
% antlion  Tune PID gains [Kp,Ki,Kd] via Ant Lion Optimizer
%
%   sys  = your state‐space or transfer‐function plant
%   [bestKp,bestKi,bestKd] = antlion(sys)

  %% ALO parameters
  nAnt     = 20;          
  Max_iter = 100;
  dim = 3;
  lb       = [0   0   0];  
  ub       = [10 5 10];  

  %% Run Ant Lion Optimizer
  %bestGains = runALO(error, nAnt, Max_iter, lb, ub);
  %bestKp = bestGains(1);
  %bestKi = bestGains(2);
  %bestKd = bestGains(3);
  %fprintf('Optimized gains: Kp=%.4f, Ki=%.4f, Kd=%.4f\n', ...
  %        bestKp, bestKi, bestKd);

   % Initialization
  antlions = rand(nAnt,dim) .* (ub - lb) + lb;
  ants     = zeros(nAnt, dim);
  fitAL    = inf(nAnt,1);
  
  % Evaluate initial fitness
  for i = 1:nAnt
      fitAL(i) = error;
  end
  elite = antlions(1,:);  % Initial elite antlion
  bestScore = fitAL(1);
  % Main loop
  for iter = 1:Max_iter
      % Update elite antlion
      [currBest, idx] = min(fitAL);
      if currBest < bestScore
          elite = antlions(idx,:);
          bestScore = currBest;
      end
      % Adaptive narrowing boundaries
      I = 10^iter/Max_iter;
      for i = 1:nAnt
          % Roulette wheel selection
          selectedAL = antlions(RouletteWheelSelection(1./(fitAL + eps)), :);
          % Random walk around selectedAL and elite
          RW1 = createRandomWalk(iter, Max_iter, lb, ub);
          RW2 = createRandomWalk(iter, Max_iter, lb, ub);
          ants(i,:) = (RW1 + RW2) / 2;
          % Bounds check
          ants(i,:) = max(min(ants(i,:), ub), lb);
      end
      % Evaluate ants
      fitAnts = inf(nAnt,1);
      for i = 1:nAnt
          fitAnts(i) = error;
      end
      % Merge and select next gen
      allPop = [antlions; ants];
      allFit = [fitAL; fitAnts];
      [allFit, idx] = sort(allFit);
      antlions = allPop(idx(1:nAnt), :);
      fitAL    = allFit(1:nAnt);
  end
  bestKp = elite(1); bestKi = elite(2); bestKd = elite(3);
end

%% Helper: Random walk (normalized)
function RW = createRandomWalk(iter, Max_iter, lb, ub)
    steps = 2*(rand(1,Max_iter)>0.5) - 1;
    walk = cumsum(steps);
    walk = (walk - min(walk)) / max(1e-6, max(walk) - min(walk)); % normalized
    RW = lb + walk(iter) .* (ub - lb);
end

%% Helper: Roulette Wheel
function idx = RouletteWheelSelection(probabilities)
    C = cumsum(probabilities / sum(probabilities));
    r = rand;
    idx = find(C >= r, 1, 'first');
end



%function bestGains = runALO(error, nAnt, Max_iter, lb, ub)
%  dim      = numel(lb);
%  antlions = rand(nAnt,dim).*(ub-lb)+lb;
%  ants      = zeros(nAnt,dim);
%  fitAL     = zeros(nAnt,1);
%
%  % Evaluate initial fitness
%  for i=1:nAnt
%    fitAL(i) = error;
%  end
%
%  for iter=1:Max_iter
%    % Roulette wheel selection
%    invFit = 1./(fitAL+eps);
%    P      = invFit/sum(invFit);
%    C      = cumsum(P);
%
%    % Move ants
%    for i=1:nAnt
%      r   = rand;
%      sel = find(C>=r,1);
%      AL  = antlions(sel,:);    % 1×3
%
%      RW = zeros(1,dim);
%      for d=1:dim
%        RW(d) = randomWalk(iter,Max_iter, lb(d), ub(d));
%      end
%
%      ants(i,:) = max(min(AL+RW, ub), lb);
%    end
%
%    % Evaluate ants
%    fitAnts = zeros(nAnt,1);
%    for i=1:nAnt
%      fitAnts(i) = error;
%    end
%
%    % Combine and select next generation antlions
%    allPop   = [antlions; ants];
%    allFit   = [fitAL; fitAnts];
%    [allFit, idx] = sort(allFit);
%    antlions = allPop(idx(1:nAnt), :);
%    fitAL    = allFit(1:nAnt);
%  end
%
%  bestGains = antlions(1,:);
%end
%
%
%function val = randomWalk(iter, Max_iter, lb, ub)
%  steps = 2*(rand(1,Max_iter)>0.5)-1;
%  walk  = cumsum(steps);
%  mn    = min(walk); mx = max(walk);
%  if mx>mn
%    normWalk = (walk-mn)/(mx-mn);
%  else
%    normWalk = zeros(size(walk));
%  end
%  val = lb + normWalk(iter)*(ub-lb);
%end

== matlab function rendezvous_optimization_ALO/Deputy Spacecraft/Guidance and Control/Control/Translational Controller/MATLAB Function ==
  data: Fb input; Fb_scaled output; in_min input; in_max input; out_min input; out_max input
function Fb_scaled = scaleForceLinear(Fb, in_min, in_max, out_min, out_max)
%SCALEFORCELINEAR Linearly scales an input force to a specified output range.
%
% Inputs:
%   Fb       - Input force (scalar or vector)
%   in_min   - Minimum expected input (e.g., -20)
%   in_max   - Maximum expected input (e.g., 20)
%   out_min  - Minimum output value (e.g., -0.05)
%   out_max  - Maximum output value (e.g., 0.05)
%
% Output:
%   Fb_scaled - Linearly mapped output value in [out_min, out_max]

Fb_scaled = ((Fb - in_min) / (in_max - in_min)) * (out_max - out_min) + out_min;

end

== matlab function rendezvous_optimization_ALO/Deputy Spacecraft/Guidance and Control/Control/Translational Controller/Outer Controller-y/Controller-2/MATLAB Function ==
  settings: updateMethod=DISCRETE
  data: bestKi output; bestKp output; bestKd output; error input
function [bestKi,bestKp,bestKd] = antlion(error)
% antlion  Tune PID gains [Kp,Ki,Kd] via Ant Lion Optimizer
%
%   sys  = your state‐space or transfer‐function plant
%   [bestKp,bestKi,bestKd] = antlion(sys)

  %% ALO parameters
  nAnt     = 20;          
  Max_iter = 100;
  dim = 3;
  lb       = [0   0   0];  
  ub       = [30 20 30];  

  %% Run Ant Lion Optimizer
  %bestGains = runALO(error, nAnt, Max_iter, lb, ub);
  %bestKp = bestGains(1);
  %bestKi = bestGains(2);
  %bestKd = bestGains(3);
  %fprintf('Optimized gains: Kp=%.4f, Ki=%.4f, Kd=%.4f\n', ...
  %        bestKp, bestKi, bestKd);

   % Initialization
  antlions = rand(nAnt,dim) .* (ub - lb) + lb;
  ants     = zeros(nAnt, dim);
  fitAL    = inf(nAnt,1);
  
  % Evaluate initial fitness
  for i = 1:nAnt
      fitAL(i) = error;
  end
  elite = antlions(1,:);  % Initial elite antlion
  bestScore = fitAL(1);
  % Main loop
  for iter = 1:Max_iter
      % Update elite antlion
      [currBest, idx] = min(fitAL);
      if currBest < bestScore
          elite = antlions(idx,:);
          bestScore = currBest;
      end
      % Adaptive narrowing boundaries
      I = 10^iter/Max_iter;
      for i = 1:nAnt
          % Roulette wheel selection
          selectedAL = antlions(RouletteWheelSelection(1./(fitAL + eps)), :);
          % Random walk around selectedAL and elite
          RW1 = createRandomWalk(iter, Max_iter, lb, ub);
          RW2 = createRandomWalk(iter, Max_iter, lb, ub);
          ants(i,:) = (RW1 + RW2) / 2;
          % Bounds check
          ants(i,:) = max(min(ants(i,:), ub), lb);
      end
      % Evaluate ants
      fitAnts = inf(nAnt,1);
      for i = 1:nAnt
          fitAnts(i) = error;
      end
      % Merge and select next gen
      allPop = [antlions; ants];
      allFit = [fitAL; fitAnts];
      [allFit, idx] = sort(allFit);
      antlions = allPop(idx(1:nAnt), :);
      fitAL    = allFit(1:nAnt);
  end
  bestKp = elite(1); bestKi = elite(2); bestKd = elite(3);
end

%% Helper: Random walk (normalized)
function RW = createRandomWalk(iter, Max_iter, lb, ub)
    steps = 2*(rand(1,Max_iter)>0.5) - 1;
    walk = cumsum(steps);
    walk = (walk - min(walk)) / max(1e-6, max(walk) - min(walk)); % normalized
    RW = lb + walk(iter) .* (ub - lb);
end

%% Helper: Roulette Wheel
function idx = RouletteWheelSelection(probabilities)
    C = cumsum(probabilities / sum(probabilities));
    r = rand;
    idx = find(C >= r, 1, 'first');
end



%function bestGains = runALO(error, nAnt, Max_iter, lb, ub)
%  dim      = numel(lb);
%  antlions = rand(nAnt,dim).*(ub-lb)+lb;
%  ants      = zeros(nAnt,dim);
%  fitAL     = zeros(nAnt,1);
%
%  % Evaluate initial fitness
%  for i=1:nAnt
%    fitAL(i) = error;
%  end
%
%  for iter=1:Max_iter
%    % Roulette wheel selection
%    invFit = 1./(fitAL+eps);
%    P      = invFit/sum(invFit);
%    C      = cumsum(P);
%
%    % Move ants
%    for i=1:nAnt
%      r   = rand;
%      sel = find(C>=r,1);
%      AL  = antlions(sel,:);    % 1×3
%
%      RW = zeros(1,dim);
%      for d=1:dim
%        RW(d) = randomWalk(iter,Max_iter, lb(d), ub(d));
%      end
%
%      ants(i,:) = max(min(AL+RW, ub), lb);
%    end
%
%    % Evaluate ants
%    fitAnts = zeros(nAnt,1);
%    for i=1:nAnt
%      fitAnts(i) = error;
%    end
%
%    % Combine and select next generation antlions
%    allPop   = [antlions; ants];
%    allFit   = [fitAL; fitAnts];
%    [allFit, idx] = sort(allFit);
%    antlions = allPop(idx(1:nAnt), :);
%    fitAL    = allFit(1:nAnt);
%  end
%
%  bestGains = antlions(1,:);
%end
%
%
%function val = randomWalk(iter, Max_iter, lb, ub)
%  steps = 2*(rand(1,Max_iter)>0.5)-1;
%  walk  = cumsum(steps);
%  mn    = min(walk); mx = max(walk);
%  if mx>mn
%    normWalk = (walk-mn)/(mx-mn);
%  else
%    normWalk = zeros(size(walk));
%  end
%  val = lb + normWalk(iter)*(ub-lb);
%end
